simulink model "end_point_filter"  (R2016b)
settings: Solver=FixedStepDiscrete  StartTime=0.0  StopTime=10  FixedStep=0.002  RelTol=1e-3
values from neighbouring files (symbols this model uses):
  rate_limit = 0.4    [init.m]
libraries: visionanalysis x3
settings Model: Creator=gaoxiao  LastModifiedBy=root
settings OptimizationCC: DefaultParameterBehavior=Inlined  ZeroExternalMemoryAtStartup=off
settings DebuggingCC: ParameterTunabilityLossMsg=error
settings RTWCC: SystemTargetFile=ert.tlc  GenCodeOnly=on  GenerateMakefile=off  TemplateMakefile=RTW.MSVCBuild  Description=Create Visual C/C++ Solution File for Embedded Coder  GenerateReport=on  IncludeHyperlinkInReport=on  LaunchReport=on  TargetLang=C++  GenerateTraceInfo=on  GenerateTraceReport=on  GenerateTraceReportSl=on  GenerateTraceReportSf=on  GenerateTraceReportEml=on  GenerateWebview=on  GenerateCodeMetricsReport=on
settings CodeAppCC: ForceParamTrailComments=on  OperatorAnnotations=on  SimulinkDataObjDesc=on  SFDataObjDesc=on  MATLABFcnDesc=on  InsertBlockDesc=on  MATLABSourceComments=on
settings ERTTargetCC: TargetLangStandard=C++03 (ISO)  GenerateSampleERTMain=on  MultiInstanceERTCode=on  CodeInterfacePackaging=C++ class  InlinedParameterPlacement=NonHierarchical  RootIOFormat=Structure reference  ERTCustomFileTemplate=example_file_process.tlc  ERTFilePackagingFormat=Compact

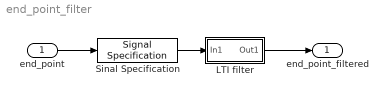
== system end_point_filter ==
  end_point : Inport  PortDimensions=3
  "LTI filter " : Subsystem
  Sinal Specification : SignalSpecification  OutDataTypeStr=double  Dimensions=3
  end_point_filtered : Outport  PortDimensions=3
  wires:
  end_point/1 -> Sinal Specification/1
  Sinal Specification/1 -> "LTI filter "/1(In1)
  "LTI filter "/1(Out1) -> end_point_filtered/1

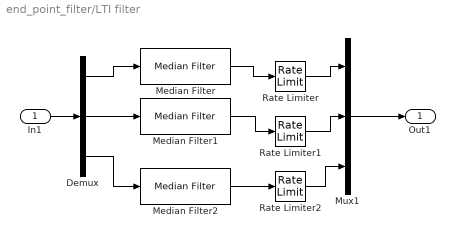
== system end_point_filter/LTI filter  ==
  In1 : Inport  PortDimensions=3
  Demux : Demux  Outputs=3
  Median Filter : visionanalysis/Median Filter  nghbood=[5 3]  outSize=Same as input port I  padType=Symmetric  padSrc=Specify via dialog  padVal=0  roundingMode=Floor  overflowMode=off
  Median Filter1 : visionanalysis/Median Filter  nghbood=[5 3]  outSize=Same as input port I  padType=Symmetric  padSrc=Specify via dialog  padVal=0  roundingMode=Floor  overflowMode=off
  Median Filter2 : visionanalysis/Median Filter  nghbood=[5 3]  outSize=Same as input port I  padType=Symmetric  padSrc=Specify via dialog  padVal=0  roundingMode=Floor  overflowMode=off
  Mux1 : Mux  Inputs=3
  Rate Limiter : RateLimiter  RisingSlewLimit=rate_limit  FallingSlewLimit=-rate_limit  SampleTimeMode=inherited
  Rate Limiter1 : RateLimiter  RisingSlewLimit=rate_limit  FallingSlewLimit=-rate_limit  SampleTimeMode=inherited
  Rate Limiter2 : RateLimiter  RisingSlewLimit=rate_limit  FallingSlewLimit=-rate_limit  SampleTimeMode=inherited
  Out1 : Outport  PortDimensions=3
  wires:
  Median Filter/1 -> Rate Limiter/1
  Median Filter1/1 -> Rate Limiter1/1
  Demux/2 -> Median Filter1/1
  Mux1/1 -> Out1/1
  In1/1 -> Demux/1
  Demux/1 -> Median Filter/1
  Rate Limiter/1 -> Mux1/1
  Rate Limiter1/1 -> Mux1/2
  Demux/3 -> Median Filter2/1
  Median Filter2/1 -> Rate Limiter2/1
  Rate Limiter2/1 -> Mux1/3
